simulink model "simulink_graph"  (R2019b)
settings: Solver=VariableStepAuto  StartTime=0.0  StopTime=5  RelTol=1e-3
settings Model: Creator=Shiwei Pan  LastModifiedBy=Shiwei Pan

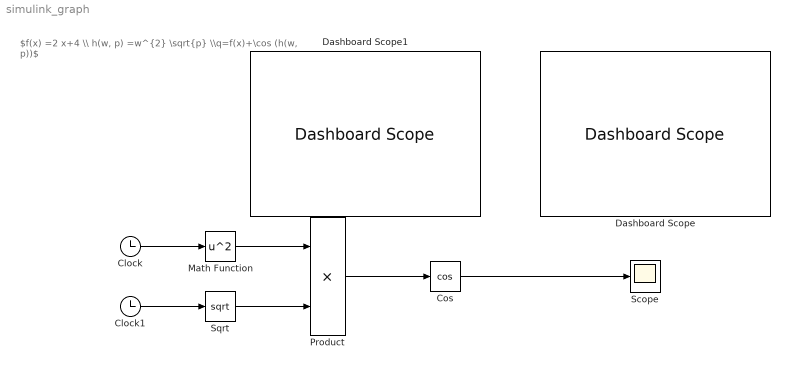
== system simulink_graph ==
  note: $f(x) =2 x+4 \\ h(w, p) =w^{2} \sqrt{p} \\q=f(x)+\cos (h(w, p))$
  Clock : Clock
  Clock1 : Clock
  Cos : Trigonometry  Operator=cos
  Dashboard Scope : DashboardScope
  Dashboard Scope1 : DashboardScope
  Math Function : Math  Operator=square  SignedPower=off  SaturateOnIntegerOverflow=on
  Product : Product
  Scope : Scope
  Sqrt : Sqrt  SaturateOnIntegerOverflow=on
  wires:
  Clock1/1 -> Sqrt/1
  Math Function/1 -> Product/1
  Sqrt/1 -> Product/2
  Product/1 -> Cos/1
  Clock/1 -> Math Function/1
  Cos/1 -> Scope/1
